simulink model "model_5LinkWalking_NODS"  (R2022b)
settings: Solver=VariableStepAuto  StartTime=0.0  StopTime=Tf  FixedStep=1e-5  MaxStep=1e-3  RelTol=1e-12  AbsTol=1e-8
values from neighbouring files (symbols this model uses):
  dq0 = [ocl_traj.simout(N,6); ocl_traj.simout(N,7); ocl_traj.simout(N,8); ocl_traj.simout(N,9); ocl_traj.simout(N,10)]    [run_walking_simulation.m]    (also in run_walking_simulation_parallel.m; search_delta_bar_parallel.m)
  gains = [K_p,K_d,K_p,K_d,K_p,K_d,K_p,K_d,K_p,K_d]    [main.m]
  init_flag = [-1; 0; ocl_traj.x_sw(1); init_t_mode_change; alpha_ref(1); 0; y_g_curr]    [run_walking_simulation.m]
  Initial_state = [q0;dq0]    [run_walking_simulation.m]    (also in run_walking_simulation_parallel.m; search_delta_bar_parallel.m)
  inputs_ref = [step_alpha_ref, step_inputs_ref]    [run_walking_simulation.m]
  joint_angles_ref = [ocl_traj.time, ocl_traj.simout, alpha_ref]    [run_walking_simulation.m]    (also in run_walking_simulation_parallel.m; search_delta_bar_parallel.m)
  landing_ref = [landing_traj.time, landing_traj.simout, alpha_ref_landing]    [run_walking_simulation.m]    (also in run_walking_simulation_parallel.m; search_delta_bar_parallel.m)
  param = [params.m1; params.m2; params.m5; params.l1; params.l2; params.l5; params.g; params.I1; params.I2; params.I5; params.r_k; params.r_h; params.k_ba; params.phi_h0; params.phi_k0]    [main.m]    (also in run_walking_simulation.m; run_walking_simulation_parallel.m)
  q0 = [ocl_traj.simout(N,1); ocl_traj.simout(N,2); ocl_traj.simout(N,3); ocl_traj.simout(N,4); ocl_traj.simout(N,5)]    [run_walking_simulation.m]    (also in run_walking_simulation_parallel.m; search_delta_bar_parallel.m)
  sample_time = 0.001    [run_walking_simulation.m]    (also in run_walking_simulation_parallel.m; search_delta_bar_parallel.m)
undefined symbols (not defined in the file or in its folder): uneven_terrain
libraries: simulink x2
(part 2 of 2)

== matlab function model_5LinkWalking_NODS/Feedback_ff_controller/Feedback_ff_controller ==
  settings: updateMethod=DISCRETE
  data: t input; X input; U output; des_theta output; des_theta_alpha output; flag_des_theta_not_defined output; param input; joint_angles_ref input; inputs_ref input; landing_ref input; gains input; flag input; x1_prev input; x1_prev output
function [U, des_theta, des_theta_alpha, flag_des_theta_not_defined, x1_prev] = fcn(t, X, param, joint_angles_ref, inputs_ref, landing_ref, gains,  flag, x1_prev)
coder.extrinsic('quadprog');
coder.extrinsic('sparse')

%% variables (absolute angles)
th1 = X(1);
th2 = X(2);
th3 = X(3);
th4 = X(4);
th5 = X(5);

dth1 = X(6);
dth2 = X(7);
dth3 = X(8);
dth4 = X(9);
dth5 = X(10);

q = [th1;th2;th3;th4;th5];
dq = [dth1;dth2;dth3;dth4;dth5];

%% Parameters

m1 = param(1);
m2 = param(2);
m3 = m2;
m4 = m1;
m5 = param(3);

l1 = param(4);
l2 = param(5);
l5 = param(6);
l3 = l2;
l4 = l1;

gravi = param(7);
I1 = param(8);
I2 = param(9);
I5 = param(10);
I3 = I1;
I4 = I2;

r_k = param(11);
r_h = param(12);
k_ba = param(13);
phi_h0 = param(14);
phi_k0 = param(15);

%% flags
f_impact = flag(1); % indicates which stance phase it is
foot = flag(2); % location of the stance foot
foot_prev = flag(3); % previous location of the stance foot
t_mode_change = flag(4); % time stamp when the mode change happens (TD or LO)
alpha_TD = flag(5); % lift off location of CoM when it happened
f_alpha_ob = flag(6); % alpha is out of bounds flag

%% Inertia Matrix
MM = MM_matrix(X,param);

%% Centrifugal force · Coriolis force Vector
CC = zeros(5,1);

CC(1, 1) = - (dth2^2*l1*l3*m3*sin(th2 + th3))/2 - dth2^2*l1*l3*m4*sin(th2 + th3) - (dth3^2*l1*l3*m3*sin(th2 + th3))/2 - dth3^2*l1*l3*m4*sin(th2 + th3) - (dth2^2*l1*l5*m5*sin(th2 + th5))/2 - (dth3^2*l2*l4*m4*sin(th3 + th4))/2 - (dth4^2*l2*l4*m4*sin(th3 + th4))/2 - (dth5^2*l1*l5*m5*sin(th2 + th5))/2 - (dth2^2*l1*l2*m2*sin(th2))/2 - dth2^2*l1*l2*m3*sin(th2) - dth2^2*l1*l2*m4*sin(th2) - dth2^2*l1*l2*m5*sin(th2) - (dth3^2*l2*l3*m3*sin(th3))/2 - dth3^2*l2*l3*m4*sin(th3) - (dth4^2*l3*l4*m4*sin(th4))/2 - (dth5^2*l2*l5*m5*sin(th5))/2 - (dth2^2*l1*l4*m4*sin(th2 + th3 + th4))/2 - (dth3^2*l1*l4*m4*sin(th2 + th3 + th4))/2 - (dth4^2*l1*l4*m4*sin(th2 + th3 + th4))/2 - dth1*dth2*l1*l3*m3*sin(th2 + th3) - 2*dth1*dth2*l1*l3*m4*sin(th2 + th3) - dth1*dth3*l1*l3*m3*sin(th2 + th3) - 2*dth1*dth3*l1*l3*m4*sin(th2 + th3) - dth2*dth3*l1*l3*m3*sin(th2 + th3) - 2*dth2*dth3*l1*l3*m4*sin(th2 + th3) - dth1*dth2*l1*l5*m5*sin(th2 + th5) - dth1*dth3*l2*l4*m4*sin(th3 + th4) - dth1*dth4*l2*l4*m4*sin(th3 + th4) - dth2*dth3*l2*l4*m4*sin(th3 + th4) - dth2*dth4*l2*l4*m4*sin(th3 + th4) - dth1*dth5*l1*l5*m5*sin(th2 + th5) - dth3*dth4*l2*l4*m4*sin(th3 + th4) - dth2*dth5*l1*l5*m5*sin(th2 + th5) - dth1*dth2*l1*l2*m2*sin(th2) - 2*dth1*dth2*l1*l2*m3*sin(th2) - 2*dth1*dth2*l1*l2*m4*sin(th2) - 2*dth1*dth2*l1*l2*m5*sin(th2) - dth1*dth3*l2*l3*m3*sin(th3) - 2*dth1*dth3*l2*l3*m4*sin(th3) - dth2*dth3*l2*l3*m3*sin(th3) - 2*dth2*dth3*l2*l3*m4*sin(th3) - dth1*dth4*l3*l4*m4*sin(th4) - dth2*dth4*l3*l4*m4*sin(th4) - dth3*dth4*l3*l4*m4*sin(th4) - dth1*dth5*l2*l5*m5*sin(th5) - dth2*dth5*l2*l5*m5*sin(th5) - dth1*dth2*l1*l4*m4*sin(th2 + th3 + th4) - dth1*dth3*l1*l4*m4*sin(th2 + th3 + th4) - dth1*dth4*l1*l4*m4*sin(th2 + th3 + th4) - dth2*dth3*l1*l4*m4*sin(th2 + th3 + th4) - dth2*dth4*l1*l4*m4*sin(th2 + th3 + th4) - dth3*dth4*l1*l4*m4*sin(th2 + th3 + th4);
CC(2, 1) = (dth1^2*l1*l3*m3*sin(th2 + th3))/2 + dth1^2*l1*l3*m4*sin(th2 + th3) + (dth1^2*l1*l5*m5*sin(th2 + th5))/2 - (dth3^2*l2*l4*m4*sin(th3 + th4))/2 - (dth4^2*l2*l4*m4*sin(th3 + th4))/2 + (dth1^2*l1*l2*m2*sin(th2))/2 + dth1^2*l1*l2*m3*sin(th2) + dth1^2*l1*l2*m4*sin(th2) + dth1^2*l1*l2*m5*sin(th2) - (dth3^2*l2*l3*m3*sin(th3))/2 - dth3^2*l2*l3*m4*sin(th3) - (dth4^2*l3*l4*m4*sin(th4))/2 - (dth5^2*l2*l5*m5*sin(th5))/2 + (dth1^2*l1*l4*m4*sin(th2 + th3 + th4))/2 - dth1*dth3*l2*l4*m4*sin(th3 + th4) - dth1*dth4*l2*l4*m4*sin(th3 + th4) - dth2*dth3*l2*l4*m4*sin(th3 + th4) - dth2*dth4*l2*l4*m4*sin(th3 + th4) - dth3*dth4*l2*l4*m4*sin(th3 + th4) - dth1*dth3*l2*l3*m3*sin(th3) - 2*dth1*dth3*l2*l3*m4*sin(th3) - dth2*dth3*l2*l3*m3*sin(th3) - 2*dth2*dth3*l2*l3*m4*sin(th3) - dth1*dth4*l3*l4*m4*sin(th4) - dth2*dth4*l3*l4*m4*sin(th4) - dth3*dth4*l3*l4*m4*sin(th4) - dth1*dth5*l2*l5*m5*sin(th5) - dth2*dth5*l2*l5*m5*sin(th5);
CC(3, 1) = (dth1^2*l1*l3*m3*sin(th2 + th3))/2 + dth1^2*l1*l3*m4*sin(th2 + th3) + (dth1^2*l2*l4*m4*sin(th3 + th4))/2 + (dth2^2*l2*l4*m4*sin(th3 + th4))/2 + (dth1^2*l2*l3*m3*sin(th3))/2 + dth1^2*l2*l3*m4*sin(th3) + (dth2^2*l2*l3*m3*sin(th3))/2 + dth2^2*l2*l3*m4*sin(th3) - (dth4^2*l3*l4*m4*sin(th4))/2 + (dth1^2*l1*l4*m4*sin(th2 + th3 + th4))/2 + dth1*dth2*l2*l4*m4*sin(th3 + th4) + dth1*dth2*l2*l3*m3*sin(th3) + 2*dth1*dth2*l2*l3*m4*sin(th3) - dth1*dth4*l3*l4*m4*sin(th4) - dth2*dth4*l3*l4*m4*sin(th4) - dth3*dth4*l3*l4*m4*sin(th4);
CC(4, 1) = (l4*m4*(dth1^2*l2*sin(th3 + th4) + dth2^2*l2*sin(th3 + th4) + dth1^2*l3*sin(th4) + dth2^2*l3*sin(th4) + dth3^2*l3*sin(th4) + dth1^2*l1*sin(th2 + th3 + th4) + 2*dth1*dth2*l2*sin(th3 + th4) + 2*dth1*dth2*l3*sin(th4) + 2*dth1*dth3*l3*sin(th4) + 2*dth2*dth3*l3*sin(th4)))/2;
CC(5, 1) = (l5*m5*(dth1^2*l1*sin(th2 + th5) + dth1^2*l2*sin(th5) + dth2^2*l2*sin(th5) + 2*dth1*dth2*l2*sin(th5)))/2;

%% Gravity Vector
GG = zeros(5,1);

GG(1, 1) = (m3*(l2*cos(th1 + th2) + l1*cos(th1) + (l3*cos(th1 + th2 + th3))/2) + m5*(l2*cos(th1 + th2) + l1*cos(th1) + (l5*cos(th1 + th2 + th5))/2) + m2*((l2*cos(th1 + th2))/2 + l1*cos(th1)) + m4*((l4*cos(th1 + th2 + th3 + th4))/2 + l2*cos(th1 + th2) + l1*cos(th1) + l3*cos(th1 + th2 + th3)) + (l1*m1*cos(th1))/2)*gravi;
GG(2, 1) = (m3*(l2*cos(th1 + th2) + (l3*cos(th1 + th2 + th3))/2) + m5*(l2*cos(th1 + th2) + (l5*cos(th1 + th2 + th5))/2) + m4*((l4*cos(th1 + th2 + th3 + th4))/2 + l2*cos(th1 + th2) + l3*cos(th1 + th2 + th3)) + (l2*m2*cos(th1 + th2))/2)*gravi;
GG(3, 1) = (m4*((l4*cos(th1 + th2 + th3 + th4))/2 + l3*cos(th1 + th2 + th3)) + (l3*m3*cos(th1 + th2 + th3))/2)*gravi;
GG(4, 1) = ((l4*m4*cos(th1 + th2 + th3 + th4))/2)*gravi;
GG(5, 1) = ((l5*m5*cos(th1 + th2 + th5))/2)*gravi;

%% input torques mapping matrix
S = [
    0,0,0,0;
    1,0,0,0;
    0,1,0,0;
    0,0,1,0;
    0,-1,0,1;];

%% Calculating the biarticular muscle torques

% Calculating the knee and hip angles
% We meed wrapTo2Pi() because some angles increase to inf due to the reset
% function eg. th1 and th5. here also X(i) is used because i usually used
% relative angles for this calculation.

phi_h_st = mod(X(5) - pi, 2*pi); % angle between torso and stance thigh
phi_k_st = mod(pi - X(2), 2*pi); % angle between stance thigh and shank
phi_h_sw = mod(X(5) - X(3), 2*pi); % angle between torso and swing thigh
phi_k_sw = mod(X(4) - pi,2 *pi); % angle between swing thigh and shank

% Calculating the elongation in the springs
delta_l_st = r_h*(phi_h_st - phi_h0) - r_k*(phi_k_st - phi_k0); % elongation of BA in stance leg [m]
delta_l_sw = r_h*(phi_h_sw - phi_h0) - r_k*(phi_k_sw - phi_k0); % elongation of BA in swing leg [m]

% torques due to BA in stance leg
tau_st = [
    0;
    -k_ba*delta_l_st*r_k;
    0;
    0;
    -k_ba*delta_l_st*r_h];

% torques due to BA in swing leg
tau_sw = [
    0;
    0;
    k_ba*delta_l_sw*r_h;
    k_ba*delta_l_sw*r_k;
    -k_ba*delta_l_sw*r_h];

%% Trajectories from OpenOCL
time_ref = joint_angles_ref(:,1);

th1_ref = joint_angles_ref(:,2);
th2_ref = joint_angles_ref(:,3);
th3_ref = joint_angles_ref(:,4);
th4_ref = joint_angles_ref(:,5);
th5_ref = joint_angles_ref(:,6);

dth1_ref = joint_angles_ref(:,7);
dth2_ref = joint_angles_ref(:,8);
dth3_ref = joint_angles_ref(:,9);
dth4_ref = joint_angles_ref(:,10);
dth5_ref = joint_angles_ref(:,11);

alpha_ref = joint_angles_ref(:,12);

% fully actuated system
% u1_ref = inputs_ref(:,1);
% u2_ref = inputs_ref(:,2);
% u3_ref = inputs_ref(:,3);
% u4_ref = inputs_ref(:,4);
% u5_ref = inputs_ref(:,5);

% under actuated system
inputs_time_ref = inputs_ref(:,1);
u2_ref = inputs_ref(:,2);
u3_ref = inputs_ref(:,3);
u4_ref = inputs_ref(:,4);
u5_ref = inputs_ref(:,5);

t_curr_step = t - t_mode_change; % timer for the current step, relative to the LO or TD time

alpha = pi - (2*th1 + th2)/2;

if t_curr_step <= time_ref(end)
    % if the current time is within the ref. traj. time
    
    th1_des = interp1(time_ref, th1_ref, t_curr_step);
    th2_des = interp1(time_ref, th2_ref, t_curr_step);
    th3_des = interp1(time_ref, th3_ref, t_curr_step);
    th4_des = interp1(time_ref, th4_ref, t_curr_step);
    th5_des = interp1(time_ref, th5_ref, t_curr_step);
    
    dth1_des = interp1(time_ref, dth1_ref, t_curr_step);
    dth2_des = interp1(time_ref, dth2_ref, t_curr_step);
    dth3_des = interp1(time_ref, dth3_ref, t_curr_step);
    dth4_des = interp1(time_ref, dth4_ref, t_curr_step);
    dth5_des = interp1(time_ref, dth5_ref, t_curr_step);

    u2_des = interp1(inputs_time_ref, u2_ref, t_curr_step);
    u3_des = interp1(inputs_time_ref, u3_ref, t_curr_step);
    u4_des = interp1(inputs_time_ref, u4_ref, t_curr_step);
    u5_des = interp1(inputs_time_ref, u5_ref, t_curr_step);
else
    % if the current time has passed the ref. traj. time
    
    th1_des = th1_ref(end);
    th2_des = th2_ref(end);
    th3_des = th3_ref(end);
    th4_des = th4_ref(end);
    th5_des = th5_ref(end);
    
    dth1_des = dth1;
    dth2_des = dth2;
    dth3_des = dth3;
    dth4_des = dth4;
    dth5_des = dth5;
        
    u2_des = 0;
    u3_des = 0;
    u4_des = 0;
    u5_des = 0;
    
%     u1_des = u1_ref(end);
%     u2_des = u1_ref(end);
%     u3_des = u1_ref(end);
%     u4_des = u1_ref(end);
%     u5_des = u1_ref(end);

end

%% prev alpha is out of bounds controller v1
flag_landing = 0; % to check when the landing reference is activated

if f_alpha_ob == 0
    % reference wrt virtual stance leg angle alpha
    th1_des_alpha = interp1(alpha_ref, th1_ref, alpha);
    th2_des_alpha = interp1(alpha_ref, th2_ref, alpha);
    th3_des_alpha = interp1(alpha_ref, th3_ref, alpha);
    th4_des_alpha = interp1(alpha_ref, th4_ref, alpha);
    th5_des_alpha = interp1(alpha_ref, th5_ref, alpha);
    
    dth1_des_alpha = interp1(alpha_ref, dth1_ref, alpha);
    dth2_des_alpha = interp1(alpha_ref, dth2_ref, alpha);
    dth3_des_alpha = interp1(alpha_ref, dth3_ref, alpha);
    dth4_des_alpha = interp1(alpha_ref, dth4_ref, alpha);
    dth5_des_alpha = interp1(alpha_ref, dth5_ref, alpha);
    
    if alpha > alpha_ref(end)
%         th1_des_alpha = th1_ref(end);
%         th2_des_alpha = th2_ref(end);
%         th3_des_alpha = th3_ref(end);
%         th4_des_alpha = th4_ref(end);
%         th5_des_alpha = th5_ref(end);
%         
%         dth1_des_alpha = dth1;
%         dth2_des_alpha = dth2;
%         dth3_des_alpha = dth3;
%         dth4_des_alpha = dth4;
%         dth5_des_alpha = dth5;
        
        %%%%%% landing ref
        %%%%%% %%%%%%%%%%%%%%%%%%%%%%%%%%%%%%%%%%%%%%%%%%%%%%%%%
        flag_landing = 1;
        
        th1_ref_landing = landing_ref(:,2);
        th2_ref_landing = landing_ref(:,3);
        th3_ref_landing = landing_ref(:,4);
        th4_ref_landing = landing_ref(:,5);
        th5_ref_landing = landing_ref(:,6);
        
        dth1_ref_landing = landing_ref(:,7);
        dth2_ref_landing = landing_ref(:,8);
        dth3_ref_landing = landing_ref(:,9);
        dth4_ref_landing = landing_ref(:,10);
        dth5_ref_landing = landing_ref(:,11);
        
        alpha_ref_landing = landing_ref(:,12);
        
        th1_des_alpha = interp1(alpha_ref_landing, th1_ref_landing, alpha);
        th2_des_alpha = interp1(alpha_ref_landing, th2_ref_landing, alpha);
        th3_des_alpha = interp1(alpha_ref_landing, th3_ref_landing, alpha);
        th4_des_alpha = interp1(alpha_ref_landing, th4_ref_landing, alpha);
        th5_des_alpha = interp1(alpha_ref_landing, th5_ref_landing, alpha);
        
        dth1_des_alpha = interp1(alpha_ref_landing, dth1_ref_landing, alpha);
        dth2_des_alpha = interp1(alpha_ref_landing, dth2_ref_landing, alpha);
        dth3_des_alpha = interp1(alpha_ref_landing, dth3_ref_landing, alpha);
        dth4_des_alpha = interp1(alpha_ref_landing, dth4_ref_landing, alpha);
        dth5_des_alpha = interp1(alpha_ref_landing, dth5_ref_landing, alpha);
        %%%%%%%%%%%%%%%%%%%%%%%%%%%%%%%%%%%%%%%%%%%%%%%%%%%%%%%%%%%%
    end
    
else
    % f_alpha_ob == 1
    alpha_merge = alpha_ref(12); % alpha when the modified alpha should merge with alpha
    
    if alpha < alpha_merge
        a = (alpha_ref(1) - alpha_TD)/(alpha_TD - alpha_merge);
        b = -a*alpha_merge;
        
        alpha_mod = alpha + a*alpha + b;
        
        th1_des_alpha = interp1(alpha_ref, th1_ref, alpha_mod);
        th2_des_alpha = interp1(alpha_ref, th2_ref, alpha_mod);
        th3_des_alpha = interp1(alpha_ref, th3_ref, alpha_mod);
        th4_des_alpha = interp1(alpha_ref, th4_ref, alpha_mod);
        th5_des_alpha = interp1(alpha_ref, th5_ref, alpha_mod);
        
        dth1_des_alpha = interp1(alpha_ref, dth1_ref, alpha_mod);
        dth2_des_alpha = interp1(alpha_ref, dth2_ref, alpha_mod);
        dth3_des_alpha = interp1(alpha_ref, dth3_ref, alpha_mod);
        dth4_des_alpha = interp1(alpha_ref, dth4_ref, alpha_mod);
        dth5_des_alpha = interp1(alpha_ref, dth5_ref, alpha_mod);
        
    elseif alpha <= alpha_ref(end)
        th1_des_alpha = interp1(alpha_ref, th1_ref, alpha);
        th2_des_alpha = interp1(alpha_ref, th2_ref, alpha);
        th3_des_alpha = interp1(alpha_ref, th3_ref, alpha);
        th4_des_alpha = interp1(alpha_ref, th4_ref, alpha);
        th5_des_alpha = interp1(alpha_ref, th5_ref, alpha);
        
        dth1_des_alpha = interp1(alpha_ref, dth1_ref, alpha);
        dth2_des_alpha = interp1(alpha_ref, dth2_ref, alpha);
        dth3_des_alpha = interp1(alpha_ref, dth3_ref, alpha);
        dth4_des_alpha = interp1(alpha_ref, dth4_ref, alpha);
        dth5_des_alpha = interp1(alpha_ref, dth5_ref, alpha);
        
    else
        % alpha > alpha_ref(end)
        
%         th1_des_alpha = th1_ref(end);
%         th2_des_alpha = th2_ref(end);
%         th3_des_alpha = th3_ref(end);
%         th4_des_alpha = th4_ref(end);
%         th5_des_alpha = th5_ref(end);
%         
%         dth1_des_alpha = dth1;
%         dth2_des_alpha = dth2;
%         dth3_des_alpha = dth3;
%         dth4_des_alpha = dth4;
%         dth5_des_alpha = dth5;
        
        %%%%%% landing ref
        %%%%%% %%%%%%%%%%%%%%%%%%%%%%%%%%%%%%%%%%%%%%%%%%%%%%%%%
        flag_landing = 1;
        
        th1_ref_landing = landing_ref(:,2);
        th2_ref_landing = landing_ref(:,3);
        th3_ref_landing = landing_ref(:,4);
        th4_ref_landing = landing_ref(:,5);
        th5_ref_landing = landing_ref(:,6);
        
        dth1_ref_landing = landing_ref(:,7);
        dth2_ref_landing = landing_ref(:,8);
        dth3_ref_landing = landing_ref(:,9);
        dth4_ref_landing = landing_ref(:,10);
        dth5_ref_landing = landing_ref(:,11);
        
        alpha_ref_landing = landing_ref(:,12);
        
        th1_des_alpha = interp1(alpha_ref_landing, th1_ref_landing, alpha);
        th2_des_alpha = interp1(alpha_ref_landing, th2_ref_landing, alpha);
        th3_des_alpha = interp1(alpha_ref_landing, th3_ref_landing, alpha);
        th4_des_alpha = interp1(alpha_ref_landing, th4_ref_landing, alpha);
        th5_des_alpha = interp1(alpha_ref_landing, th5_ref_landing, alpha);
        
        dth1_des_alpha = interp1(alpha_ref_landing, dth1_ref_landing, alpha);
        dth2_des_alpha = interp1(alpha_ref_landing, dth2_ref_landing, alpha);
        dth3_des_alpha = interp1(alpha_ref_landing, dth3_ref_landing, alpha);
        dth4_des_alpha = interp1(alpha_ref_landing, dth4_ref_landing, alpha);
        dth5_des_alpha = interp1(alpha_ref_landing, dth5_ref_landing, alpha);
        %%%%%%%%%%%%%%%%%%%%%%%%%%%%%%%%%%%%%%%%%%%%%%%%%%%%%%%%%%%%
    end    
end

%%
flag_des_theta_not_defined = 0;
if isnan(th1_des_alpha)
    flag_des_theta_not_defined = 1;
    K_P1 = gains(1); % gain for CoM control
    K_D1 = gains(2); % gain for CoM control
end


%% Controller Gains
K_P1 = gains(1); % gain for CoM control
K_D1 = gains(2); % gain for CoM control
K_P2 = gains(3); % gain for CoM control
K_D2 = gains(4); % gain for CoM control
K_P3 = gains(5); % gain for CoM control
K_D3 = gains(6); % gain for CoM control
K_P4 = gains(7); % gain for CoM control
K_D4 = gains(8); % gain for CoM control
K_P5 = gains(9); % gain for CoM control
K_D5 = gains(10); % gain for CoM control

%% Feedback linearization controller

% constant task space matrix
T = [
    0,1,0,0,0;
    0,0,1,0,0;
    0,0,0,1,0;
    0,0,0,0,1];

%% Output Feedback Control

%%%%% alpha ref %%%%%
y_alpha = [th2; th3; th4; th5] - [th2_des_alpha; th3_des_alpha; th4_des_alpha; th5_des_alpha];
dy_alpha = [dth2; dth3; dth4; dth5] - [dth2_des_alpha; dth3_des_alpha; dth4_des_alpha; dth5_des_alpha];

K_p = [
    K_P2, 0, 0, 0;
    0, K_P3, 0, 0;
    0, 0, K_P4, 0;
    0, 0, 0, K_P5];

K_d = [
    K_D2, 0, 0, 0;
    0, K_D3, 0, 0;
    0, 0, K_D4, 0;
    0, 0, 0, K_D5];

v_alpha = -K_p*y_alpha - K_d*dy_alpha;

% u_alpha_fb = inv(T*inv(MM)*S)*(v_alpha + T*inv(MM)*(CC+GG));

% controller with BA muscles
u_alpha_fb = inv(T*inv(MM)*S)*(v_alpha + T*inv(MM)*(CC+GG-tau_st-tau_sw));

% u_alpha_ff = [u2_des; u3_des; u4_des; u5_des];
%%%%%%%%%%%%%%%%%%%%%

U = zeros(5,1);

U(1) = 0;
U(2) = u_alpha_fb(1);
U(3) = u_alpha_fb(2);
U(4) = u_alpha_fb(3);
U(5) = u_alpha_fb(4);

U(1) = 0;
U(2) = sign(U(2))*min(abs(U(2)), 200);
U(3) = sign(U(3))*min(abs(U(3)), 200);
U(4) = sign(U(4))*min(abs(U(4)), 200);
U(5) = sign(U(5))*min(abs(U(5)), 200);

%%
des_theta = [th1_des; th2_des; th3_des; th4_des; th5_des; dth1_des; dth2_des; dth3_des; dth4_des; dth5_des];
des_theta_alpha = [th1_des_alpha; th2_des_alpha; th3_des_alpha; th4_des_alpha; th5_des_alpha;
    dth1_des_alpha; dth2_des_alpha; dth3_des_alpha; dth4_des_alpha; dth5_des_alpha; flag_landing];

end

== matlab function model_5LinkWalking_NODS/Model dynamics/Mode Changer/Mode Changer 5Link ==
  data: X_minus input; flag output; flag_minus input; param input; uneven_terrain input; joint_angles_ref input; X_reset output; time input
function [flag, X_reset]  = fcn(X_minus, flag_minus, param, uneven_terrain, joint_angles_ref, time)

%% variables

th1 = X_minus(1);
th2 = X_minus(2);
th3 = X_minus(3);
th4 = X_minus(4);
th5 = X_minus(5);

dth1 = X_minus(6);
dth2 = X_minus(7);
dth3 = X_minus(8);
dth4 = X_minus(9);
dth5 = X_minus(10);

q = [th1;th2;th3;th4;th5];
dq = [dth1;dth2;dth3;dth4;dth5];

%% parameters

m1 = param(1);
m2 = param(2);
m3 = m2;
m4 = m1;
m5 = param(3);

l1 = param(4);
l2 = param(5);
l5 = param(6);
l3 = l2;
l4 = l1;

gravi = param(7);
I1 = param(8);
I2 = param(9);
I5 = param(10);
I3 = I1;
I4 = I2;

q_minus = [th1;th2;th3;th4;th5];
dq_minus = [dth1;dth2;dth3;dth4;dth5];

%% flags
f_impact = flag_minus(1); % indicates which stance phase it is
foot_x = flag_minus(2); % location of the stance foot
foot_x_prev = flag_minus(3); % previous location of the stance foot
t_LO = flag_minus(4); % previous location of the stance foot
alpha_TD = flag_minus(5); % x_CoM location when liftOff happens
f_alpha_ob = flag_minus(6); % alpha is out of bounds flag
foot_y = flag_minus(7); 

%% reference 
alpha_ref = joint_angles_ref(:,12);

%%
X_reset = [q_minus; dq_minus]; % dummy X_reset so that simulink doesn't give error

%% calculating the Swing foot position and velocity
Psw_tip_minus = [l1*cos(th1) + l2*cos(th1 + th2) + l3*cos(th1 + th2 + th3) + l4*cos(th1 + th2 + th3 + th4);
                 foot_y + l1*sin(th1) + l2*sin(th1 + th2) + l3*sin(th1 + th2 + th3) + l4*sin(th1 + th2 + th3 + th4)];
 
J_Psw_tip_minus = [- l4*sin(th1 + th2 + th3 + th4) - l2*sin(th1 + th2) - l1*sin(th1) - l3*sin(th1 + th2 + th3), - l4*sin(th1 + th2 + th3 + th4) - l2*sin(th1 + th2) - l3*sin(th1 + th2 + th3), - l4*sin(th1 + th2 + th3 + th4) - l3*sin(th1 + th2 + th3), -l4*sin(th1 + th2 + th3 + th4), 0;
                   l4*cos(th1 + th2 + th3 + th4) + l2*cos(th1 + th2) + l1*cos(th1) + l3*cos(th1 + th2 + th3),   l4*cos(th1 + th2 + th3 + th4) + l2*cos(th1 + th2) + l3*cos(th1 + th2 + th3),   l4*cos(th1 + th2 + th3 + th4) + l3*cos(th1 + th2 + th3),  l4*cos(th1 + th2 + th3 + th4), 0];

dPsw_tip_minus = J_Psw_tip_minus*dq_minus;

%% calculating the current height of the ground (uneven ground)
x_sw = Psw_tip_minus(1,1);
x_g = uneven_terrain.track_start:uneven_terrain.dist_step_size:uneven_terrain.track_end;
y_g = uneven_terrain.y_g_curr;
y_g_curr = interp1(x_g, y_g, foot_x + x_sw);

%%

% if f_SS == 1 && Psw_tip_minus(2,1) <= 0.005 && dPsw_tip_minus(2,1) < -0.5
if Psw_tip_minus(2,1) <= y_g_curr && dPsw_tip_minus(2,1) < -0.005
    % touchdown (impact)
    f_impact = 1;
    foot_x_prev = foot_x; % saving the old foot location
    foot_x = foot_x_prev + Psw_tip_minus(1,1); % calculating the new foots location
    foot_y = y_g_curr; % new stance foot height
           
    % Impact mapによる衝突後の状態の計算
    MM_minus = MM_matrix(X_minus,param);
    dq_after = (eye(5)-inv(MM_minus)*J_Psw_tip_minus'*inv(J_Psw_tip_minus*inv(MM_minus)*J_Psw_tip_minus')*J_Psw_tip_minus)*dq_minus;
    
    %
    th1_after = q_minus(4,1) + q_minus(3,1) + q_minus(2,1) + q_minus(1,1) - pi; % th1 becomes th4
    th2_after = - q_minus(4,1); % th2 becomes th3
    th3_after = - q_minus(3,1); % th3 becomes th2
    th4_after = - q_minus(2,1); % th4 becomes th1
    %th5_after = q_minus(5,1) - q_minus(3,1) + pi;
    th5_after = q_minus(1,1) + q_minus(2,1) + q_minus(5,1) - (th1_after + th2_after);
    
    % constraining angles to pi 2pi
    th1_after = mod(th1_after, 2*pi);
    th2_after = mod(th2_after, 2*pi);
    th3_after = mod(th3_after, 2*pi) - 2*pi;
    th4_after = mod(th4_after, 2*pi);
    th5_after = th5_after - 2*pi;
    
    q_after = [th1_after; th2_after; th3_after; th4_after; th5_after]; % this is where the switching happens
    
    dth1_after = dq_after(4,1) + dq_after(3,1) + dq_after(2,1) + dq_after(1,1); % th1 becomes th4
    dth2_after = - dq_after(4,1); % th2 becomes th3
    dth3_after = - dq_after(3,1); % th3 becomes th2
    dth4_after = - dq_after(2,1); % th4 becomes th1
    dth5_after = dq_after(5,1) - dq_after(3,1);
    
    % Reset state if the f_ss change from 1 to 0 (from single stance to
    % double stance)
    X_reset = [q_after; dth1_after; dth2_after; dth3_after; dth4_after; dth5_after];
    
    alpha_TD = pi - (2*th1_after + th2_after)/2;
    t_LO = time;
    
    % check is alpha is out of bounds and raise the flag is so
    if alpha_TD < alpha_ref(1)
        f_alpha_ob = 1;
    else
        f_alpha_ob = 0;
    end
        
elseif f_impact == 1 && Psw_tip_minus(2,1) > y_g_curr + 0.01
    f_impact = -1;

end

flag = [f_impact; foot_x; foot_x_prev; t_LO; alpha_TD; f_alpha_ob; foot_y];

== matlab function model_5LinkWalking_NODS/Model dynamics/STOP system when dx_CoM<=0/MATLAB Function2 ==
  data: X input; param input; flag input; flag_zCoM_pos output; flag_xCoM_vel output; flag_th2 output; flag_th4 output; flag_5 output
function [flag_zCoM_pos, flag_xCoM_vel, flag_th2, flag_th4, flag_5] = fcn(X,param, flag)

%% variables
th1 = X(1);
th2 = X(2);
th3 = X(3);
th4 = X(4);
th5 = X(5);

dth1 = X(6);
dth2 = X(7);
dth3 = X(8);
dth4 = X(9);
dth5 = X(10);

q = [th1;th2;th3;th4;th5];
dq = [dth1;dth2;dth3;dth4;dth5];

%% parameters

m1 = param(1);
m2 = param(2);
m3 = m2;
m4 = m1;
m5 = param(3);

l1 = param(4);
l2 = param(5);
l5 = param(6);
l3 = l2;
l4 = l1;

gravi = param(7);
I1 = param(8);
I2 = param(9);
I5 = param(10);
I3 = I1;
I4 = I2;

k_s = param(11);
r_k = param(12);
r_b = param(13);

%% flags
f_SS = flag(1); % indicates which stance phase it is
foot = flag(2); % location of the stance foot
foot_prev = flag(3); % previous location of the stance foot

%% CoM calculation
% CoM = [xG, zG, dxG, dzG, ddxG, ddzG];
CoM = calculate_com(X, param, flag, [0;0;0;0;0]); % calculation the CoM location

xG = CoM(1);
zG = CoM(2);
dxG = CoM(3);
dzG = CoM(4);

%%

% flag_zCoM_pos: if z_CoM drops or rises above certain value
flag_zCoM_pos = 0;
if zG >= 1.5
    flag_zCoM_pos = 1;
elseif zG <= 0.7
    flag_zCoM_pos = 1;
end

% flag_xCoM_vel
flag_xCoM_vel = 0;
if dxG <= 0
    flag_xCoM_vel = 1;
end

% flag_th2
flag_th2 = 0;
if mod(th2,2*pi) <= 0
    flag_th2 = 1;
end

% flag_th4
flag_th4 = 0;
if mod(th4,2*pi) >= 0
%     flag_th4 = 1;
end

% flag_th5
flag_5 = 0;
if foot > 0
    flag_5 = 0;
end
